simulink model "sys_v2"  (R2024b)
settings: Solver=FixedStepAuto  StartTime=0.0  StopTime=10  FixedStep=0.001  RelTol=1e-3
values from neighbouring files (symbols this model uses):
  c = 2/5    (= 0.4)    [analysis.m]
  g = 9.8    [analysis.m]
  Ip = 1.8 * 10^-4    (= 0.00018)    [analysis.m]
  kd = 2*(1+c)/(g*alpha)    (= 0.285714285714)    [analysis.m]
  kp = (1+c)/(g*alpha^2)    (= 0.142857142857)    [analysis.m]
  m = 0.01838    [analysis.m]
libraries: simulink x2, slpidlib x1
settings Model: Creator=Jacob  LastModifiedBy=Jacob

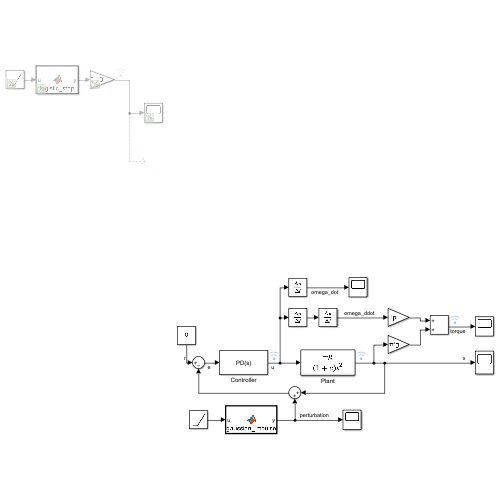
[thumbnail: Simulink's stored preview of the top-level diagram]
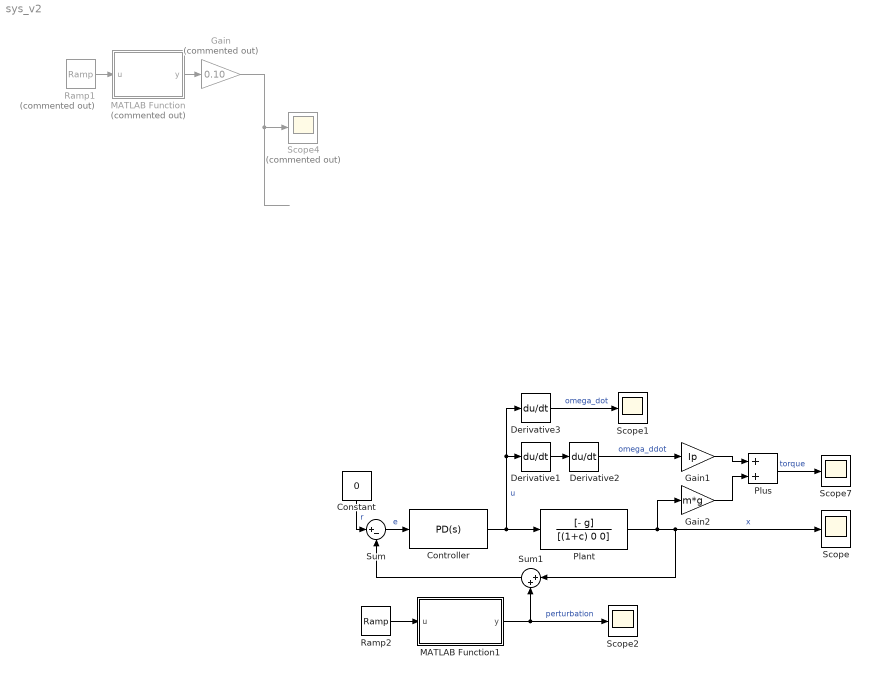
== system sys_v2 ==
  Constant : Constant  Value=0
  Controller : slpidlib/PID Controller  Controller=PD  Form=Parallel  TimeDomain=Continuous-time  UseExternalTs=off  SampleTime=-1  IntegratorMethod=Forward Euler  FilterMethod=Forward Euler  ControllerParametersSource=internal  P=-kp  I=0  UseKiTs=off  D=-kd  UseExternalDerivativeSource=off  N=1000  UseFilter=on  TunerSelectOption=Transfer Function Based (PID Tuner App)  InitialConditionSource=internal  InitialConditionForIntegrator=0  InitialConditionForFilter=0  DifferentiatorICPrevScaledInput=0  ExternalReset=none  TrackingMode=off  Kt=1  LimitOutput=off  SatLimitsSource=internal  UpperSaturationLimit=inf  LowerSaturationLimit=-inf  LinearizeAsGain=on  AntiWindupMode=none  Kb=1  LimitIntegrator=off  UpperIntegratorSaturationLimit=inf  LowerIntegratorSaturationLimit=-inf  POutMin=[]  POutMax=[]  IOutMin=[]  IOutMax=[]  DOutMin=[]  DOutMax=[]  NOutMin=[]  NOutMax=[]  SumOutMin=[]  SumOutMax=[]  SaturationOutMin=[]  SaturationOutMax=[]  PParamMin=[]  PParamMax=[]  IParamMin=[]  IParamMax=[]  DParamMin=[]  DParamMax=[]  NParamMin=[]  NParamMax=[]  KbParamMin=[]  KbParamMax=[]  KtParamMin=[]  KtParamMax=[]  KbOutMin=[]  KbOutMax=[]  KtOutMin=[]  KtOutMax=[]  IntegratorOutMin=[]  IntegratorOutMax=[]  FilterOutMin=[]  FilterOutMax=[]  SumI1OutMin=[]  SumI1OutMax=[]  SumI2OutMin=[]  SumI2OutMax=[]  SumI3OutMin=[]  SumI3OutMax=[]  SumI4OutMin=[]  SumI4OutMax=[]  SumDOutMin=[]  SumDOutMax=[]  DifferentiatorOutMin=[]  DifferentiatorOutMax=[]  FilterDiffOutCoefMin=[]  FilterDiffOutCoefMax=[]  ReciprocalOutMin=[]  ReciprocalOutMax=[]  SumDenOutMin=[]  SumDenOutMax=[]  SumNumOutMin=[]  SumNumOutMax=[]  DivideOutMin=[]  DivideOutMax=[]  UdiffTsProdOutMin=[]  UdiffTsProdOutMax=[]  NTsProdOutMin=[]  NTsProdOutMax=[]  UintegralTsProdOutMin=[]  UintegralTsProdOutMax=[]  UngainTsProdOutMin=[]  UngainTsProdOutMax=[]  ClampingZeroOutDataTypeStr=Inherit: Inherit via back propagation  ClampingZeroOutMin=[]  ClampingZeroOutMax=[]  FilterDenConstantOutDataTypeStr=Inherit: Inherit via back propagation  FilterDenConstantOutMin=[]  FilterDenConstantOutMax=[]  PCopyOutDataTypeStr=Inherit: Inherit via back propagation  PCopyOutMin=[]  PCopyOutMax=[]  NCopyOutDataTypeStr=Inherit: Inherit via back propagation  NCopyOutMin=[]  NCopyOutMax=[]  IntegratorContinuousStateAttributes=''  IntegratorStateMustResolveToSignalObject=off  IntegratorRTWStateStorageClass=Auto  FilterContinuousStateAttributes=''  FilterStateMustResolveToSignalObject=off  FilterRTWStateStorageClass=Auto  ParallelPVariant=InternalParameters  IdealPVariant=Disabled  IVariant=Disabled  DVariant=InternalParameters  IntegratorVariant=Disabled  SatVariant=Disabled  AWVariant=Disabled  PCopyVariant=Disabled  TRVariant=Disabled  FdbkBlocksVariant=Forward  IdealPFdbkVariant=Disabled  SatFdbkVariant=Disabled  DerivativeFilterVariant=ContFilter  NVariant=InternalParameters  NCopyVariant=Disabled  FilterICVariant=InternalICsFilter  IntegratorICVariant=Disabled  ExternalResetVariant=Disabled  TRSumVariant=Passthrough  SumFdbkVariant=Disabled  SumVariant=Sum_PD  TsampFilterVariant=InternalTs  TsampNgainVariant=Passthrough  TsampIntegralVariant=Disabled_SignalSpec  ExternalSaturationOutDataTypeStr=Inherit: Same as second input  DerivativeSourceVariant=ErrorSignal  PreIntVariant=InternalPreInt
  Derivative1 : Derivative
  Derivative2 : Derivative
  Derivative3 : Derivative
  Gain : Gain  Commented=on  Gain=0.10
  Gain1 : Gain  Gain=Ip
  Gain2 : Gain  Gain=m*g
  MATLAB Function : MATLAB Function  Commented=on  TreatAsAtomicUnit=on
  MATLAB Function1 : MATLAB Function  TreatAsAtomicUnit=on
  Plant : TransferFcn  Numerator=[- g]  Denominator=[(1+c) 0 0]
  Plus : Sum
  Ramp1 : simulink/Sources/Ramp  Commented=on  slope=1  start=0  InitialOutput=0
  Ramp2 : simulink/Sources/Ramp  slope=1  start=0  InitialOutput=0
  Scope{,1..2,7} (4 alike) : Scope
  Scope4 : Scope  Commented=on
  Sum : Sum  Inputs=|+-
  Sum1 : Sum  Inputs=|++
  wires:
  Controller/1 -> Derivative3/1, Derivative1/1, Plant/1  "u"
  Sum/1 -> Controller/1  "e"
  Plant/1 -> Sum1/1, Scope/1, Gain2/1  "x"
  Derivative1/1 -> Derivative2/1
  Derivative2/1 -> Gain1/1  "omega_ddot"
  Gain1/1 -> Plus/1
  Gain2/1 -> Plus/2
  Plus/1 -> Scope7/1  "torque"
  MATLAB Function/1(y) -> Gain/1
  Ramp1/1 -> MATLAB Function/1(u)
  Derivative3/1 -> Scope1/1  "omega_dot"
  Gain/1 -> Scope4/1
  Constant/1 -> Sum/1  "r"
  Sum1/1 -> Sum/2
  Ramp2/1 -> MATLAB Function1/1(u)
  MATLAB Function1/1(y) -> Scope2/1, Sum1/2  "perturbation"

== matlab function sys_v2/MATLAB Function ==
  data: u input; y output
function y = logistic_step(u)
    y = 1/(1+exp(-75*u+100));
end

== matlab function sys_v2/MATLAB Function1 ==
  data: u input; y output
function y = gaussian_impulse(u)
    y = 0.1*exp(-(10*(u-1))^2);
end
